simulink model "Praktikum01Grupp09"  (R2023b)
settings: Solver=VariableStepAuto  StartTime=0.0  StopTime=128e-9  RelTol=1e-3
undefined symbols (not defined in the file): doppler, magnitude
libraries: commchan3 x2, commrflib2 x2, dspsrcs4 x1
settings Model: Creator=suttarar@hu-berlin.de

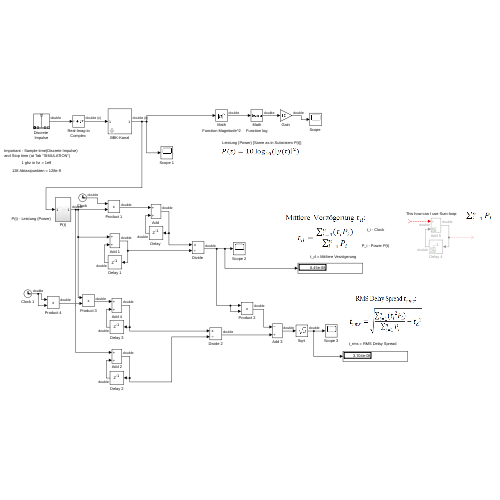
[thumbnail: Simulink's stored preview of the top-level diagram]
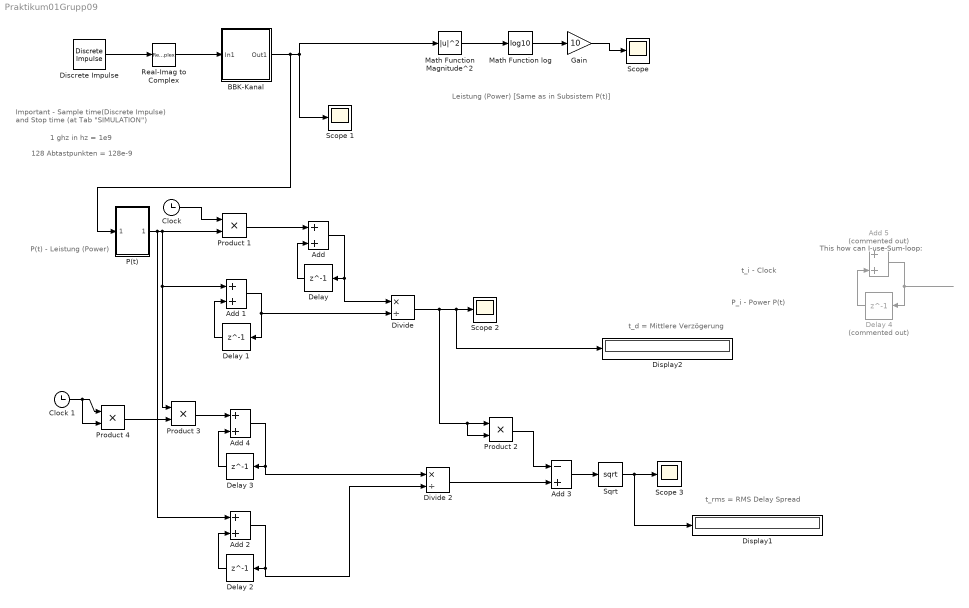
== system Praktikum01Grupp09 ==
  note: 128 Abtastpunkten = 128e-9
  note: 1 ghz in hz = 1e9
  note: Important - Sample time(Discrete Impulse)
      | and Stop time (at Tab "SIMULATION")
  note: P_i - Power P(t)
  note: t_i - Clock
  note: This how can I use Sum-loop:
  note: Leistung (Power) [Same as in Subsistem P(t)]
  note: t_rms = RMS Delay Spread
  note: t_d = Mittlere Verzögerung
  note: P(t) - Leistung (Power)
  Add {,1..2,4} (4 alike) : Sum
  Add 3 : Sum  Inputs=-+
  Add 5 : Sum  Commented=on
  BBK-Kanal : Subsystem  mask{MaxDoppler=20, PathDelays=[0 3 6 12]*1e-9, PathGains=[0 -1 -2 -4], EnableMultipath=0, PathLoss=0, FrequencyOffset=0, PhaseOffset=0, SNR=50}
      mask prompts: MaxDoppler "Dopplerverschiebung"; PathDelays "Pfadverzoergerungen"; PathGains "Pfadverstaerkungen"; EnableMultipath "SwitchBlock"; PathLoss "Pfadverlust"; FrequencyOffset "Frequenzverschiebung"; PhaseOffset "Phasenverschiebung"; SNR "AWG-Rauschen"
  "Clock " : Clock
  Clock 1 : Clock
  Delay {,1..3} (4 alike) : Delay  DelayLength=1  InitialCondition=0
  Delay 4 : Delay  Commented=on  DelayLength=1  InitialCondition=0
  Discrete Impulse : dspsrcs4/Discrete  Impulse  Delay=0  SampleTime=1/1e9  FrameSample=1  OutputFrames=off  dataType=double  isSigned=on  wordLen=16  udDataType=sfix(16)  fracBitsMode=Best precision  numFracBits=15  OutDataTypeStr=double  LastOutDataTypeStr=double
  Display1 : Display
  Display2 : Display
  "Divide " : Product  Inputs=*/
  Divide 2 : Product  Inputs=*/
  "Gain " : Gain  Gain=10
  Math Function Magnitude^2 : Math  Operator=magnitude^2
  Math Function log : Math  Operator=log10
  P(t) : Subsystem
  Product {1..4} (4 alike) : Product
  "Real-Imag to Complex " : RealImagToComplex  Input=Real
  Scope {,1..3} (4 alike) : Scope
  "Sqrt " : Sqrt
  wires:
  Discrete Impulse/1 -> "Real-Imag to Complex "/1
  "Real-Imag to Complex "/1 -> BBK-Kanal/1(In1)
  Math Function Magnitude^2/1 -> Math Function log/1
  Product 1/1 -> "Add "/1
  BBK-Kanal/1(Out1) -> P(t)/1(In1), Scope 1/1, Math Function Magnitude^2/1
  "Clock "/1 -> Product 1/1
  "Add "/1 -> "Divide "/1, "Delay "/1
  "Delay "/1 -> "Add "/2
  Add 1/1 -> Delay 1/1, "Divide "/2
  Delay 1/1 -> Add 1/2
  Add 2/1 -> Divide 2/2, Delay 2/1
  Delay 2/1 -> Add 2/2
  "Divide "/1 -> Product 2/2, Product 2/1, Display2/1, Scope 2/1
  Add 3/1 -> "Sqrt "/1
  Product 2/1 -> Add 3/1
  Divide 2/1 -> Add 3/2
  Delay 3/1 -> Add 4/2
  Add 4/1 -> Divide 2/1, Delay 3/1
  Product 3/1 -> Add 4/1
  P(t)/1(Out1) -> Add 2/1, Product 3/1, Add 1/1, Product 1/2
  Clock 1/1 -> Product 4/2, Product 4/1
  Product 4/1 -> Product 3/2
  "Sqrt "/1 -> Display1/1, Scope 3/1
  Math Function log/1 -> "Gain "/1
  "Gain "/1 -> "Scope "/1
  Delay 4/1 -> Add 5/2
  Add 5/1 -> Delay 4/1
  ? -> Add 5/1

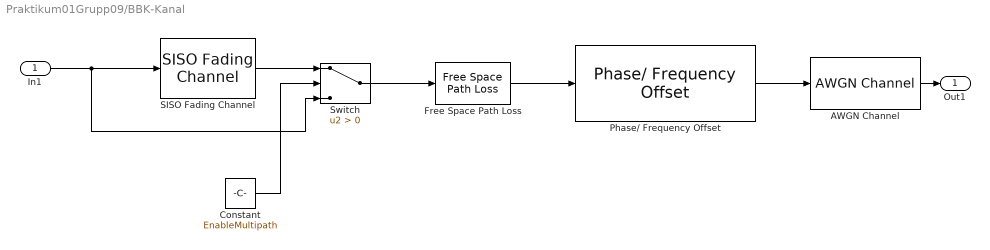
== system Praktikum01Grupp09/BBK-Kanal ==
  In1 : Inport
  AWGN Channel : commchan3/AWGN Channel  LegacyMode=off  NoiseMethod="Signal to noise ratio  (SNR)"  noiseMode="Signal to noise ratio  (SNR)"  EbNo=10  EsNo=10  SNR=SNR  BitsPerSymbol=1  SignalPower=1  SamplesPerSymbol=1  SymbolPeriod=1  VarianceSource=Parameter  Variance=1  RandomStream=Global stream  Seed=67  SimulateUsing=Code generation
  Constant : Constant  Value=EnableMultipath
  Free Space Path Loss : commrflib2/Free Space Path Loss  mode=Decibels  dB=PathLoss  d=0.100  fc=1920
  Phase/ Frequency Offset : commrflib2/Phase// Frequency Offset  phaseOffset=PhaseOffset  freqPort=off  freqOffset=FrequencyOffset
      settings: LibrarySourceBlock=|
      | commrfcorlib/Phase//
      | Frequency
      | Offset
  SISO Fading Channel : commchan3/SISO Fading Channel  InheritSampleRate=on  SampleRate=1  PathDelays=PathDelays  AveragePathGains=PathGains  NormalizePathGains=on  FadingDistribution=Rayleigh  KFactor=3  DirectPathDopplerShift=0  DirectPathInitialPhase=0  MaximumDopplerShift=MaxDoppler  DopplerSpectrum=doppler('Jakes')  RandomStream=mt19937ar with seed  Seed=73  PathGainsOutputPort=off  ChannelFilterDelayOutputPort=off  SimulateUsing=Interpreted execution  Visualization=Off  PathsForDopplerDisplay=1  SamplesToDisplay=25%
  Switch : Switch  Criteria=u2 > Threshold  SaturateOnIntegerOverflow=off  InputSameDT=off
  Out1 : Outport
  wires:
  Phase/ Frequency Offset/1 -> AWGN Channel/1
  Free Space Path Loss/1 -> Phase/ Frequency Offset/1
  AWGN Channel/1 -> Out1/1
  Switch/1 -> Free Space Path Loss/1
  SISO Fading Channel/1 -> Switch/1
  In1/1 -> Switch/3, SISO Fading Channel/1
  Constant/1 -> Switch/2

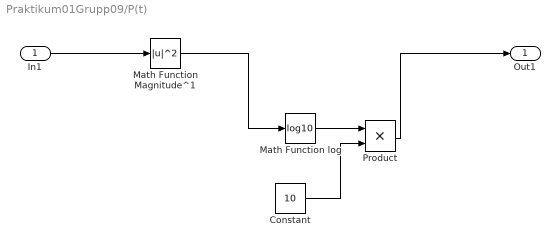
== system Praktikum01Grupp09/P(t) ==
  In1 : Inport
  "Constant " : Constant  Value=10
  Math Function Magnitude^1 : Math  Operator=magnitude^2
  Math Function log : Math  Operator=log10
  "Product " : Product
  Out1 : Outport
  wires:
  In1/1 -> Math Function Magnitude^1/1
  "Product "/1 -> Out1/1
  Math Function log/1 -> "Product "/1
  "Constant "/1 -> "Product "/2
  Math Function Magnitude^1/1 -> Math Function log/1
